simulink model "req14"  (R2019a)
settings: Solver=FixedStepAuto  StartTime=0.0  StopTime=100  RelTol=1e-3
libraries: simulink x1
settings Model: Creator=e40014285  LastModifiedBy=e40014285
settings ConfigComp: CovScope=ReferencedModels  CovHTMLOptions=-sRT=1 -sVT=0 -aTS=1 -bRG=1 -bTC=1 -hTR=0 -nFC=0 -nFD=1 -scm=1 -bcm=1 -xEv=0 -xEM=0  CovHtmlReporting=on  CovCumulativeReport=on  DVModelCoverageObjectives=EnhancedMCDC  DVTestSuiteOptimization=Auto  DVDetectOutOfBounds=on  DVReportPDFFormat=on  DVRebuildModelRepresentation=Always

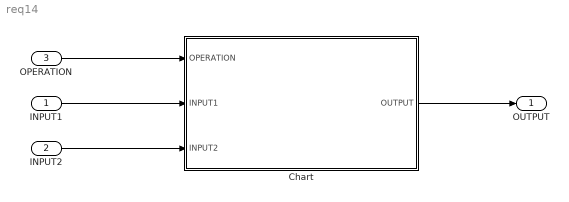
== system req14 ==
  INPUT1 : Inport
  INPUT2 : Inport  Port=2
  OPERATION : Inport  Port=3
  Chart : Stateflow chart  BlockKeywords=__PRM__SERIALIZED__DATA__:Stateflow Chart,Stateflow Diagram  TreatAsAtomicUnit=on
  OUTPUT : Outport
  wires:
  Chart/1(OUTPUT) -> OUTPUT/1
  INPUT2/1 -> Chart/3(INPUT2)
  INPUT1/1 -> Chart/2(INPUT1)
  OPERATION/1 -> Chart/1(OPERATION)

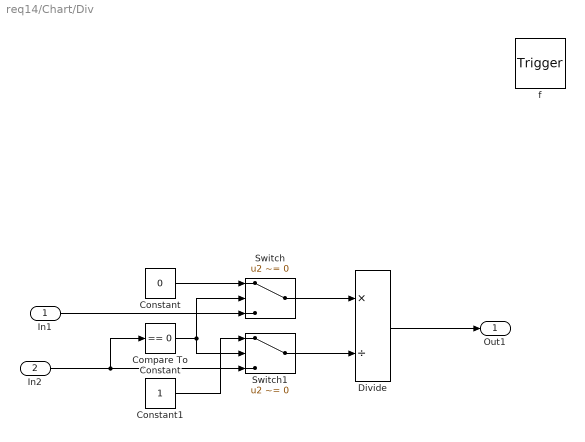
== system req14/Chart/Div ==
  In1 : Inport  OutDataTypeStr=double  PortDimensions=1
  In2 : Inport  Port=2  OutDataTypeStr=double  PortDimensions=1
  f : TriggerPort  TriggerType=function-call  VariantControl=(inherit)
      settings: CopyFcn=Stateflow.SLINSF.SimulinkMan.removeBlockPreDeleteFcn  PreDeleteFcn=Stateflow.SLINSF.SimulinkMan.unsafePredeleteFcn
  Compare To Constant : simulink/Logic and Bit Operations/Compare To Constant  relop===  const=0  OutDataTypeStr=boolean
  Constant : Constant  Value=0
  Constant1 : Constant
  Divide : Product  Inputs=*/
  Switch : Switch  Criteria=u2 ~= 0
  Switch1 : Switch  Criteria=u2 ~= 0
  Out1 : Outport
  wires:
  In1/1 -> Switch/3
  In2/1 -> Compare To Constant/1, Switch1/3
  Compare To Constant/1 -> Switch1/2, Switch/2
  Constant/1 -> Switch/1
  Switch/1 -> Divide/1
  Constant1/1 -> Switch1/1
  Switch1/1 -> Divide/2
  Divide/1 -> Out1/1

== stateflow chart req14/Chart ==
  state Addition_1_
    OUTPUT=INPUT1+INPUT2;
  state resetState
  state Out1 = Div(In1,In2) [function]
  state Subtraction_2_
    OUTPUT=INPUT1-INPUT2;
  state SubtractionModulp_3_
    OUTPUT=INPUT1-INPUT2;
  state multiplication_4_
    OUTPUT=INPUT1*INPUT2;
  state exponential_5_
    loc1=uint32(INPUT1);
    loc2=uint32(INPUT2);
    OUTPUT=double(loc1^loc2);
  state division_6_
    OUTPUT=Div(INPUT1,INPUT2);
  state divisionmodulo_7_
    OUTPUT=rem(INPUT1,INPUT2);
  (default) -> Addition_1_
  Addition_1_ -> resetState : [OPERATION==2||OPERATION==3||OPERATION==4 ...
      | ||OPERATION==5||OPERATION==6||OPERATION==7]
  resetState -> Addition_1_ [order 1] : [OPERATION==1]
  Subtraction_2_ -> resetState : [OPERATION==1||OPERATION==3||OPERATION==4 ...
      | ||OPERATION==5||OPERATION==6||OPERATION==7]
  resetState -> Subtraction_2_ [order 7] : [OPERATION==2]
  SubtractionModulp_3_ -> resetState : [OPERATION==1||OPERATION==2||OPERATION==4 ...
      | ||OPERATION==5||OPERATION==6||OPERATION==7]
  resetState -> SubtractionModulp_3_ [order 6] : [OPERATION==3]
  multiplication_4_ -> resetState : [OPERATION==1||OPERATION==2||OPERATION==3 ...
      | ||OPERATION==5||OPERATION==6||OPERATION==7]
  resetState -> multiplication_4_ [order 5] : [OPERATION==4]
  exponential_5_ -> resetState : [OPERATION==1||OPERATION==2||OPERATION==3 ...
      | ||OPERATION==4||OPERATION==6||OPERATION==7]
  resetState -> exponential_5_ [order 4] : [OPERATION==5]
  division_6_ -> resetState : [OPERATION==1||OPERATION==2||OPERATION==3 ...
      | ||OPERATION==4||OPERATION==5||OPERATION==7]
  resetState -> division_6_ [order 3] : [OPERATION==6]
  divisionmodulo_7_ -> resetState : [OPERATION==1||OPERATION==2||OPERATION==3 ...
      | ||OPERATION==4||OPERATION==5||OPERATION==6]
  resetState -> divisionmodulo_7_ [order 2] : [OPERATION==7]
  data: In1 function_input double size=1; In2 function_input double size=1; Out1 function_output; OUTPUT output; OPERATION input; INPUT1 input; INPUT2 input; loc1 local; loc2 local
